simulink model "test_fed"  (R2022a)
settings: Solver=VariableStepAuto  StartTime=0.0  StopTime=10.0  RelTol=1e-3
settings Model: Creator=top1  LastModifiedBy=top1

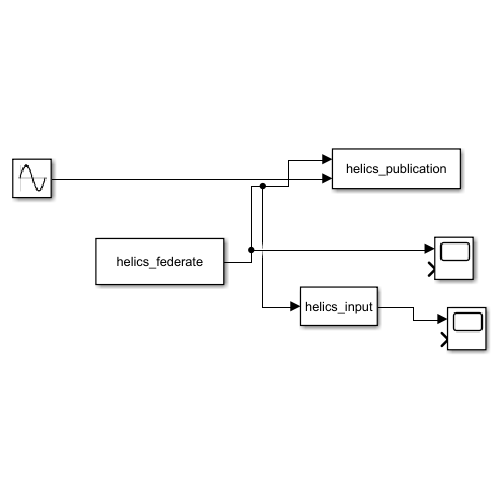
[thumbnail: Simulink's stored preview of the top-level diagram]
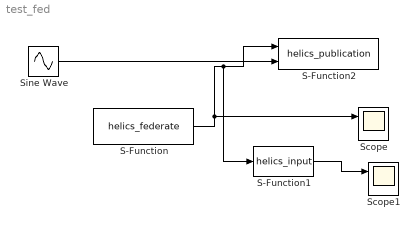
== system test_fed ==
  S-Function : S-Function  FunctionName=helics_federate  Parameters='sim_config.json'  SFunctionDeploymentMode=off  EnableBusSupport=off
  S-Function1 : S-Function  FunctionName=helics_input  Parameters=0,'output_type=double'  SFunctionDeploymentMode=off  EnableBusSupport=off
  S-Function2 : S-Function  FunctionName=helics_publication  Parameters=0,'input_size=1'  SFunctionDeploymentMode=off  EnableBusSupport=off
  Scope : Scope  NumInputPorts=2
  Scope1 : Scope  NumInputPorts=2
  Sine Wave : Sin  Amplitude=3  SampleTime=0
  wires:
  S-Function/1 -> S-Function2/1, S-Function1/1, Scope/1
  Sine Wave/1 -> S-Function2/2
  S-Function1/1 -> Scope1/1
